simulink model "sensor_model_simulink"  (R2021a)
settings: Solver=FixedStepAuto  StartTime=0.0  StopTime=inf  FixedStep=0.1  RelTol=1e-3
StartFcn:
  | addpath([pwd, '\init']);
  | init_simulink
settings Model: EnablePacing=on  Creator=samue  LastModifiedBy=samue

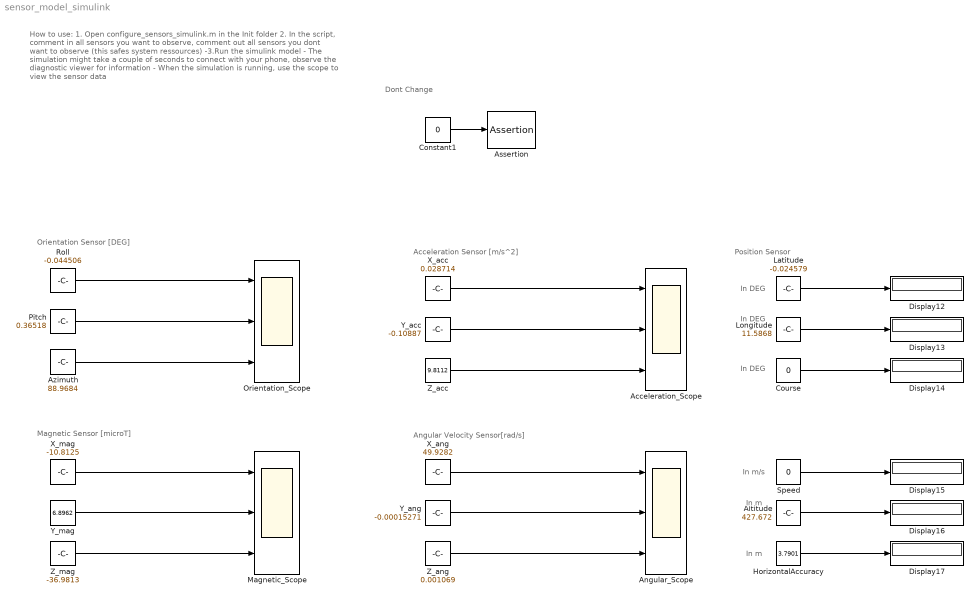
== system sensor_model_simulink ==
  note: How to use:
      |
      | 1. Open configure_sensors_simulink.m in the Init folder
      |
      | 2. In the script, comment in all sensors you want to observe, comment out all sensors you dont want to observe (this safes system ressources)
      |
      | -3.Run the simulink model
      | - The simulation might take a couple of seconds to connect with your phone, observe the diagnostic viewer for information
      | - When the simulation is running, use the scope to view the sensor data
  note: In DEG
  note: Dont Change
  note: Orientation Sensor [DEG]
  note: Magnetic Sensor [microT]
  note: Acceleration Sensor [m/s^2]
  note: Angular Velocity Sensor[rad/s]
  note: Position Sensor
  note: In DEG
  note: In DEG
  note: In m/s
  note: In m
  note: In m
  Acceleration_Scope : Scope  NumInputPorts=3
  Altitude : Constant  Value=427.672
  Angular_Scope : Scope  NumInputPorts=3
  Assertion : Assertion  AssertionFailFcn=configure_sensors_simulink  StopWhenAssertionFail=off
  Azimuth : Constant  Value=88.9684
  Constant1 : Constant  Value=0
  Course : Constant  Value=0
  Display{12..17} (6 alike) : Display
  HorizontalAccuracy : Constant  Value=3.7901
  Latitude : Constant  Value=-0.024579
  Longitude : Constant  Value=11.5868
  Magnetic_Scope : Scope  NumInputPorts=3
  Orientation_Scope : Scope  NumInputPorts=3
  Pitch : Constant  Value=0.36518
  Roll : Constant  Value=-0.044506
  Speed : Constant  Value=0
  X_acc : Constant  Value=0.028714
  X_ang : Constant  Value=49.9282
  X_mag : Constant  Value=-10.8125
  Y_acc : Constant  Value=-0.10887
  Y_ang : Constant  Value=-0.00015271
  Y_mag : Constant  Value=6.8962
  Z_acc : Constant  Value=9.8112
  Z_ang : Constant  Value=0.001069
  Z_mag : Constant  Value=-36.9813
  wires:
  Roll/1 -> Orientation_Scope/1
  Constant1/1 -> Assertion/1
  Pitch/1 -> Orientation_Scope/2
  Azimuth/1 -> Orientation_Scope/3
  Z_mag/1 -> Magnetic_Scope/3
  Y_mag/1 -> Magnetic_Scope/2
  X_mag/1 -> Magnetic_Scope/1
  Z_acc/1 -> Acceleration_Scope/3
  Y_acc/1 -> Acceleration_Scope/2
  X_acc/1 -> Acceleration_Scope/1
  X_ang/1 -> Angular_Scope/1
  Y_ang/1 -> Angular_Scope/2
  Z_ang/1 -> Angular_Scope/3
  Latitude/1 -> Display12/1
  Longitude/1 -> Display13/1
  Course/1 -> Display14/1
  Speed/1 -> Display15/1
  Altitude/1 -> Display16/1
  HorizontalAccuracy/1 -> Display17/1
